simulink model "Waste_Classification"  (R2019a)
settings: Solver=FixedStepAuto  StartTime=0.0  StopTime=inf  FixedStep=0.002  RelTol=1e-3  EnableMultiTasking=on
undefined symbols (not defined in the file): height, HIL, left, qc_get_step_size, top, width
libraries: simulink x19, quarc_library x19
settings Model: SimulationMode=external  ExtModeTrigDuration=10000  Creator=dell  LastModifiedBy=郑怡迪
settings SolverCC: PositivePriorityOrder=on  AutoInsertRateTranBlk=on
settings RTWCC: SystemTargetFile=quarc_win64.tlc  TemplateMakefile=quarc_default_tmf  Description=QUARC Win64 Target
settings STFCustomTargetCC: TargetPreCompLibLocation=C:\PROGRA~3\QUARC\lib\2019a\win64\release  TargetLangStandard=C99 (ISO)  ConcurrentExecutionCompliant=on  SystemTargetFile=quarc_win64.tlc
settings GRTTargetCC: TargetPreCompLibLocation=C:\PROGRA~3\QUARC\lib\2019a\win64\release  ParMdlRefBuildCompliant=off  CompOptLevelCompliant=off  CombineOutputUpdateFcns=off  MatFileLogging=off  CPPClassGenCompliant=off  GRTInterface=on  UseToolchainInfoCompliant=off  ExtMode=on  ExtModeMexFile=quarc_comm

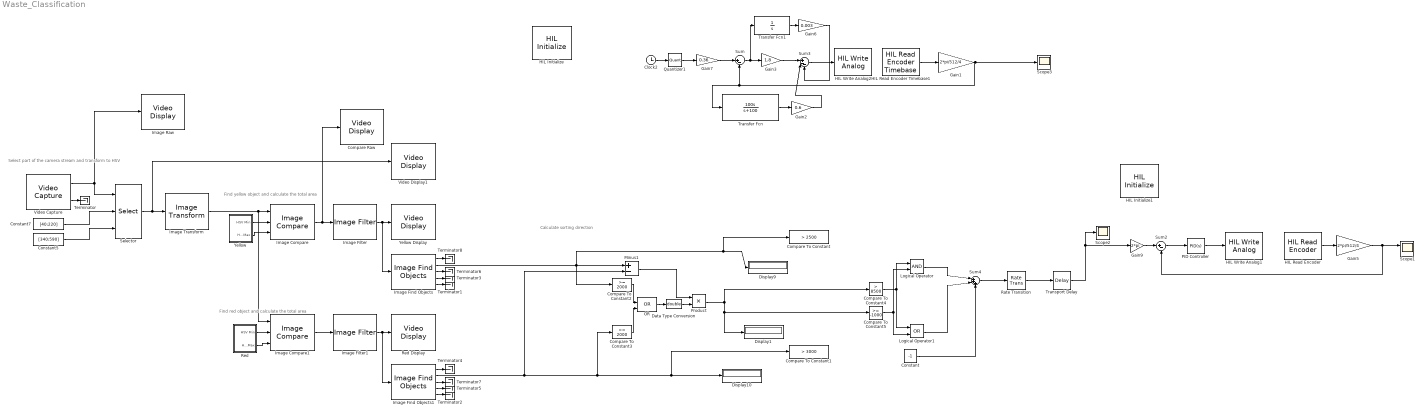
== system Waste_Classification ==
  note: Calculate sorting direction
  note: Find red object and calculate the total area
  note: Find yellow object and calculate the total area
  note: Select part of the camera stream and transform to HSV
  Clock2 : Clock
  Compare To Constant : simulink/Logic and Bit Operations/Compare To Constant  relop=>  const=2500  OutDataTypeStr=boolean
  Compare To Constant1 : simulink/Logic and Bit Operations/Compare To Constant  relop=>  const=3000  OutDataTypeStr=boolean
  Compare To Constant2 : simulink/Logic and Bit Operations/Compare To Constant  relop=>=  const=2000  OutDataTypeStr=boolean
  Compare To Constant3 : simulink/Logic and Bit Operations/Compare To Constant  relop=>=  const=2000  OutDataTypeStr=boolean
  Compare To Constant4 : simulink/Logic and Bit Operations/Compare To Constant  relop=>  const=8500  OutDataTypeStr=boolean
  Compare To Constant5 : simulink/Logic and Bit Operations/Compare To Constant  relop=>=  const=-1000  OutDataTypeStr=boolean
  Compare Raw : quarc_library/Multimedia/Video Display  Tag=slowlybeat6661/Compare Raw  sample_time=-1  use_hardware=on
  Constant : Constant  Value=-1
  Constant5 : Constant  Value=[340:590]
  Constant7 : Constant  Value=[40:220]
  Data Type Conversion : DataTypeConversion  OutDataTypeStr=double
  Display1 : Display
  Display10 : Display
  Display9 : Display
  Gain1 : Gain  Gain=2*pi/512/4
  Gain2 : Gain  Gain=0.6
  Gain3 : Gain  Gain=1.8
  Gain5 : Gain  Gain=2*pi/512/4
  Gain6 : Gain  Gain=0.003
  Gain7 : Gain  Gain=0.36
  Gain9 : Gain  Gain=2*pi
  HIL Initialize : quarc_library/Data Acquisition/Generic/Configuration/HIL Initialize  object_name=HIL-1  board_type=qube_servo2_usb  board_number=0  board_options=""  exclusive=off  active=on  hardware_clocks=[0]  clock_modes=[]  initial_clock_frequencies=[]  set_clock_params_at_start=off  set_clock_params_at_switch_in=off  set_clock_frequencies_at_start=off  set_clock_frequencies_at_switch_in=off  analog_input_channels=[0]  analog_input_configurations=[]  analog_input_maximums=3  analog_input_minimums=-3  set_analog_input_params_at_start=off  set_analog_input_params_at_switch_in=off  analog_output_channels=[0]  analog_output_maximums=15  analog_output_minimums=-15  initial_analog_outputs=[0]  final_analog_outputs=[0]  watchdog_analog_outputs=0  set_analog_output_params_at_start=off  set_analog_output_params_at_switch_in=off  set_analog_outputs_at_start=on  set_analog_outputs_at_switch_in=off  set_analog_outputs_at_terminate=on  set_analog_outputs_at_switch_out=off  set_analog_outputs_on_watchdog=on  digital_input_channels=[]  digital_output_channels=[0]  digital_output_configuration=[]  initial_digital_outputs=[1]  final_digital_outputs=[0]  watchdog_digital_outputs=[0]  set_digital_output_params_at_start=off  set_digital_output_params_at_switch_in=off  set_digital_outputs_at_start=on  set_digital_outputs_at_switch_in=off  set_digital_outputs_at_terminate=on  set_digital_outputs_at_switch_out=off  set_digital_outputs_on_watchdog=on  encoder_channels=[0:1]  quadrature=[4]  encoder_filter_frequency=[]  initial_encoder_counts=[0]  set_encoder_params_at_start=off  set_encoder_params_at_switch_in=off  set_encoder_counts_at_start=on  set_encoder_counts_at_switch_in=off  pwm_channels=[]  pwm_modes=[]  pwm_frequency=[]  pwm_configuration=[]  pwm_alignment=[]  pwm_polarity=[]  pwm_leading_deadband=[]  pwm_trailing_deadband=[]  initial_pwm_outputs=[]  final_pwm_outputs=[]  watchdog_pwm_outputs=[]  set_pwm_params_at_start=off  set_pwm_params_at_switch_in=off  set_pwm_outputs_at_start=off  set_pwm_outputs_at_switch_in=off  set_pwm_outputs_at_terminate=off  set_pwm_outputs_at_switch_out=off  set_pwm_outputs_on_watchdog=off  other_output_channels=[11000:11002]  initial_other_outputs=[0 1 0]  final_other_outputs=[1 0 0]  watchdog_other_outputs=[0 0 1]  set_other_outputs_at_start=on  set_other_outputs_at_switch_in=off  set_other_outputs_at_terminate=on  set_other_outputs_at_switch_out=off  set_other_outputs_on_watchdog=on
  HIL Initialize1 : quarc_library/Data Acquisition/Generic/Configuration/HIL Initialize  object_name=HIL-2  board_type=qube_servo2_usb  board_number=1  board_options=""  exclusive=off  active=on  hardware_clocks=[0]  clock_modes=[]  initial_clock_frequencies=[]  set_clock_params_at_start=off  set_clock_params_at_switch_in=off  set_clock_frequencies_at_start=off  set_clock_frequencies_at_switch_in=off  analog_input_channels=[0]  analog_input_configurations=[]  analog_input_maximums=3  analog_input_minimums=-3  set_analog_input_params_at_start=off  set_analog_input_params_at_switch_in=off  analog_output_channels=[0]  analog_output_maximums=15  analog_output_minimums=-15  initial_analog_outputs=[0]  final_analog_outputs=[0]  watchdog_analog_outputs=0  set_analog_output_params_at_start=off  set_analog_output_params_at_switch_in=off  set_analog_outputs_at_start=on  set_analog_outputs_at_switch_in=off  set_analog_outputs_at_terminate=on  set_analog_outputs_at_switch_out=off  set_analog_outputs_on_watchdog=on  digital_input_channels=[]  digital_output_channels=[0]  digital_output_configuration=[]  initial_digital_outputs=[1]  final_digital_outputs=[0]  watchdog_digital_outputs=[0]  set_digital_output_params_at_start=off  set_digital_output_params_at_switch_in=off  set_digital_outputs_at_start=on  set_digital_outputs_at_switch_in=off  set_digital_outputs_at_terminate=on  set_digital_outputs_at_switch_out=off  set_digital_outputs_on_watchdog=on  encoder_channels=[0:1]  quadrature=[4]  encoder_filter_frequency=[]  initial_encoder_counts=[0]  set_encoder_params_at_start=off  set_encoder_params_at_switch_in=off  set_encoder_counts_at_start=on  set_encoder_counts_at_switch_in=off  pwm_channels=[]  pwm_modes=[]  pwm_frequency=[]  pwm_configuration=[]  pwm_alignment=[]  pwm_polarity=[]  pwm_leading_deadband=[]  pwm_trailing_deadband=[]  initial_pwm_outputs=[]  final_pwm_outputs=[]  watchdog_pwm_outputs=[]  set_pwm_params_at_start=off  set_pwm_params_at_switch_in=off  set_pwm_outputs_at_start=off  set_pwm_outputs_at_switch_in=off  set_pwm_outputs_at_terminate=off  set_pwm_outputs_at_switch_out=off  set_pwm_outputs_on_watchdog=off  other_output_channels=[11000:11002]  initial_other_outputs=[0 1 0]  final_other_outputs=[1 0 0]  watchdog_other_outputs=[0 0 1]  set_other_outputs_at_start=on  set_other_outputs_at_switch_in=off  set_other_outputs_at_terminate=on  set_other_outputs_at_switch_out=off  set_other_outputs_on_watchdog=on
  HIL Read Encoder : quarc_library/Data Acquisition/Generic/Immediate I//O/HIL Read Encoder  object_name=HIL-2  channels=0  sample_time=qc_get_step_size  active=on  vector_output=off  data_type_mode=Inherit via back propagation  data_type=double
  HIL Read Encoder Timebase1 : quarc_library/Data Acquisition/Generic/Timebases/HIL Read Encoder Timebase  object_name=HIL-1  clock=0  channels=0  samples_in_buffer=max(ceil(1/qc_get_step_size), 1)  active=on  vector_output=off  data_type_mode=Inherit via back propagation  data_type=double
  HIL Write Analog1 : quarc_library/Data Acquisition/Generic/Immediate I//O/HIL Write Analog  object_name=HIL-2  channels=0  sample_time=-1  active=off  vector_input=off
  HIL Write Analog2 : quarc_library/Data Acquisition/Generic/Immediate I//O/HIL Write Analog  object_name=HIL-1  channels=0  sample_time=-1  active=off  vector_input=off
  Image Compare : quarc_library/Image Processing/Generic/Image Compare  output_type=Combined (one HxW output)  source=External input ports  r_comparison=min <= pixel and pixel <= max  r_minimum=0  r_maximum=16  g_comparison=min <= pixel and pixel <= max  g_minimum=128  g_maximum=255  b_comparison=min <= pixel and pixel <= max  b_minimum=64  b_maximum=255
      settings: SourceProductName=QUARC Targets
  Image Compare1 : quarc_library/Image Processing/Generic/Image Compare  output_type=Combined (one HxW output)  source=External input ports  r_comparison=min <= pixel and pixel <= max  r_minimum=0  r_maximum=16  g_comparison=min <= pixel and pixel <= max  g_minimum=128  g_maximum=255  b_comparison=min <= pixel and pixel <= max  b_minimum=64  b_maximum=255
      settings: SourceProductName=QUARC Targets
  Image Filter : quarc_library/Image Processing/Generic/Image Filter  filter_type=Depth hole-fill  source_of_roi=Internal dialog parameter  roi_style=[top, left, height, width]  roi=[]  maximum_roi=[]  roi_zone=Operate inside region of interest  border_type=Replicate  border_value=[0 0 0]  kernel_size=5  sigma=10  mask_size=[3 3]  kernel=int16([-2 -1 0; -1 1 1; 0 1 2])  divisor=1  offset=0  rounding=Nearest  algorithm_hint=None  threshold=100  alpha=0.9  num_frames=8  num_valid=1  gap_threshold=10  depth_threshold=255  iterations=2
      settings: AttributesFormatString=(%<filter_type>)  SourceProductName=QUARC Targets
  Image Filter1 : quarc_library/Image Processing/Generic/Image Filter  filter_type=Depth hole-fill  source_of_roi=Internal dialog parameter  roi_style=[top, left, height, width]  roi=[]  maximum_roi=[]  roi_zone=Operate inside region of interest  border_type=Replicate  border_value=[0 0 0]  kernel_size=5  sigma=10  mask_size=[3 3]  kernel=int16([-2 -1 0; -1 1 1; 0 1 2])  divisor=1  offset=0  rounding=Nearest  algorithm_hint=None  threshold=100  alpha=0.9  num_frames=8  num_valid=1  gap_threshold=10  depth_threshold=255  iterations=2
      settings: AttributesFormatString=(%<filter_type>)  SourceProductName=QUARC Targets
  Image Find Objects : quarc_library/Image Processing/Generic/Image Find Objects  num_objects=1  connectivity=4 directions (N, E, S, W)  sort_order=Sort by number of pixels  min_pixels=256  max_pixels=intmax('uint32')  largest=on  exclude_at_edges=off  variable_size=off  use_complex=off
      settings: SourceProductName=QUARC Targets
  Image Find Objects1 : quarc_library/Image Processing/Generic/Image Find Objects  num_objects=1  connectivity=4 directions (N, E, S, W)  sort_order=Sort by number of pixels  min_pixels=256  max_pixels=intmax('uint32')  largest=on  exclude_at_edges=off  variable_size=off  use_complex=off
      settings: SourceProductName=QUARC Targets
  Image Raw : quarc_library/Multimedia/Video Display  Tag=slowlybeat6661/Image Raw  sample_time=-1  use_hardware=on
  Image Transform : quarc_library/Image Processing/Generic/Image Transform  algorithm=RGB to HSV  color_theme=KRYGCBMW  min_pixel=0  max_pixel=4000
      settings: AttributesFormatString=(%<algorithm>)  SourceProductName=QUARC Targets
  Logical Operator : Logic  AllPortsSameDT=off  OutDataTypeStr=boolean
  Logical Operator1 : Logic  Operator=OR  AllPortsSameDT=off  OutDataTypeStr=boolean
  Minus1 : Sum  Inputs=+-  OutDataTypeStr=double
  OR : Logic  Operator=OR  IconShape=distinctive  AllPortsSameDT=off  OutDataTypeStr=boolean
  PID Controller : simulink/Continuous/PID Controller  Controller=PID  Form=Parallel  TimeDomain=Continuous-time  SampleTime=-1  IntegratorMethod=Forward Euler  FilterMethod=Forward Euler  ControllerParametersSource=internal  P=5  I=0.15  D=0.2  UseFilter=on  N=100  TunerSelectOption=Transfer Function Based (PID Tuner App)  InitialConditionSource=internal  InitialConditionForIntegrator=0  InitialConditionForFilter=0  DifferentiatorICPrevScaledInput=0  ExternalReset=none  TrackingMode=off  Kt=1  LimitOutput=off  UpperSaturationLimit=inf  LowerSaturationLimit=-inf  LinearizeAsGain=on  AntiWindupMode=none  Kb=1  POutMin=[]  POutMax=[]  IOutMin=[]  IOutMax=[]  DOutMin=[]  DOutMax=[]  NOutMin=[]  NOutMax=[]  SumOutMin=[]  SumOutMax=[]  SaturationOutMin=[]  SaturationOutMax=[]  PParamMin=[]  PParamMax=[]  IParamMin=[]  IParamMax=[]  DParamMin=[]  DParamMax=[]  NParamMin=[]  NParamMax=[]  KbParamMin=[]  KbParamMax=[]  KtParamMin=[]  KtParamMax=[]  KbOutMin=[]  KbOutMax=[]  KtOutMin=[]  KtOutMax=[]  IntegratorOutMin=[]  IntegratorOutMax=[]  FilterOutMin=[]  FilterOutMax=[]  SumI1OutMin=[]  SumI1OutMax=[]  SumI2OutMin=[]  SumI2OutMax=[]  SumI3OutMin=[]  SumI3OutMax=[]  SumI4OutMin=[]  SumI4OutMax=[]  SumDOutMin=[]  SumDOutMax=[]  DifferentiatorOutMin=[]  DifferentiatorOutMax=[]  FilterDiffOutCoefMin=[]  FilterDiffOutCoefMax=[]  ReciprocalOutMin=[]  ReciprocalOutMax=[]  SumDenOutMin=[]  SumDenOutMax=[]  SumNumOutMin=[]  SumNumOutMax=[]  DivideOutMin=[]  DivideOutMax=[]  IntegratorContinuousStateAttributes=''  IntegratorStateMustResolveToSignalObject=off  IntegratorRTWStateStorageClass=Auto  FilterContinuousStateAttributes=''  FilterStateMustResolveToSignalObject=off  FilterRTWStateStorageClass=Auto  ParallelPVariant=InternalParameters  IdealPVariant=Disabled  IVariant=InternalParameters  DVariant=InternalParameters  IntegratorVariant=Continuous  SatVariant=Disabled  AWVariant=Passthrough  PCopyVariant=Disabled  TRVariant=Disabled  FdbkBlocksVariant=Forward  IdealPFdbkVariant=Disabled  SatFdbkVariant=Disabled  DerivativeFilterVariant=ContFilter  NVariant=InternalParameters  NCopyVariant=Disabled  FilterICVariant=InternalICsFilter  IntegratorICVariant=InternalICs  ExternalResetVariant=Disabled  TRSumVariant=Passthrough  SumFdbkVariant=Disabled  SumVariant=Sum_PID
  Product : Product
  Quantizer1 : Quantizer
  Rate Transition : RateTransition
  Red : Subsystem
  Red Display : quarc_library/Multimedia/Video Display  Tag=slowlybeat6661/Red Display  sample_time=-1  use_hardware=on
  Scope1 : Scope  NumInputPorts=2
  Scope2 : Scope
  Scope3 : Scope
  Selector : Selector  NumberOfDimensions=3  IndexOptions=Index vector (port),Index vector (port),Select all  Indices=[1 3],1,1  OutputSizes=1,1,1
  Sum : Sum  Inputs=|+-
  Sum2 : Sum  Inputs=|+-
  Sum3 : Sum  Inputs=|+--
  Sum4 : Sum  Inputs=|+++
  Terminator{,1..8} (9 alike) : Terminator
  Transfer Fcn : TransferFcn  Numerator=[100 0]  Denominator=[1 100]
  Transfer Fcn1 : TransferFcn  Denominator=[1 0]
  Transport Delay : TransportDelay
  Video Capture : quarc_library/Multimedia/Video Capture  source=device  device=0  filename=sample_movie.mov  value=[0 0; 0 0]  resolution=640 x 480  width=640  height=480  output_format=MATLAB RGB (HxWx3)  data_type=uint8  sample_time=qc_get_step_size * ceil(0.033 / qc_get_step_size)  brightness_override=off  brightness=54.0  contrast_override=off  contrast=0.0  hue_override=off  hue=50.0  saturation_override=off  saturation=50  sharpness_override=off  sharpness=50.0  gamma_override=off  gamma=50.0  coloreffect_override=off  coloreffect=None  whitebalance_override=off  whitebalance=0.0  backlightcompensation_override=off  backlightcompensation=0.0  gain_override=off  gain=0.0  pan_override=off  pan=50.0  tilt_override=off  tilt=50.0  roll_override=off  roll=50.0  zoom_override=off  zoom=0.0  exposure_override=off  exposure=50.0  iris_override=off  iris=50.0  focus_override=off  focus=0.0
      settings: SourceProductName=QUARC Targets
  Video Display1 : quarc_library/Multimedia/Video Display  Tag=slowlybeat6661/Video Display1  sample_time=-1  use_hardware=on
  Yellow : Subsystem
  Yellow Display : quarc_library/Multimedia/Video Display  Tag=slowlybeat6661/Yellow Display  sample_time=-1  use_hardware=on
  wires:
  Gain5/1 -> Scope1/1, Sum2/2
  HIL Read Encoder/1 -> Gain5/1
  Product/1 -> Compare To Constant4/1, Compare To Constant5/1, Display1/1
  OR/1 -> Data Type Conversion/1
  Image Find Objects/1 -> Terminator8/1
  Constant7/1 -> Selector/2
  Video Capture/1 -> Image Raw/1, Selector/1
  Image Filter1/1 -> Image Find Objects1/1, Red Display/1
  Image Find Objects1/1 -> Terminator4/1
  Red/2(HSV Max) -> Image Compare1/3
  Image Find Objects1/2 -> Minus1/2, Display10/1, Compare To Constant1/1, Compare To Constant3/1
  Compare To Constant3/1 -> OR/2
  Selector/1 -> Video Display1/1, Image Transform/1
  Image Find Objects1/5 -> Terminator2/1
  Image Compare1/1 -> Image Filter1/1
  Yellow/2(HSV Max) -> Image Compare/3
  Image Compare/1 -> Image Filter/1, Compare Raw/1
  Image Find Objects/5 -> Terminator1/1
  Image Transform/1 -> Image Compare1/1, Image Compare/1
  Image Find Objects/4 -> Terminator3/1
  Image Filter/1 -> Yellow Display/1, Image Find Objects/1
  Image Find Objects1/3 -> Terminator7/1
  Video Capture/2 -> Terminator/1
  Image Find Objects/3 -> Terminator6/1
  Image Find Objects/2 -> Display9/1, Compare To Constant/1, Minus1/1, Compare To Constant2/1
  Image Find Objects1/4 -> Terminator5/1
  Data Type Conversion/1 -> Product/2
  Minus1/1 -> Product/1
  Red/1(HSV Min) -> Image Compare1/2
  Constant5/1 -> Selector/3
  Yellow/1(HSV Min) -> Image Compare/2
  Compare To Constant2/1 -> OR/1
  Compare To Constant4/1 -> Logical Operator1/1, Logical Operator/1
  Logical Operator/1 -> Sum4/1
  Logical Operator1/1 -> Sum4/2
  Constant/1 -> Sum4/3
  Sum4/1 -> Rate Transition/1
  Transport Delay/1 -> Scope2/1, Gain9/1
  Compare To Constant5/1 -> Logical Operator/2, Logical Operator1/2
  PID Controller/1 -> HIL Write Analog1/1
  Gain9/1 -> Sum2/1
  Sum2/1 -> PID Controller/1
  Gain7/1 -> Sum/1
  Quantizer1/1 -> Gain7/1
  Gain6/1 -> Sum3/3
  Clock2/1 -> Quantizer1/1
  Transfer Fcn1/1 -> Gain6/1
  Sum3/1 -> HIL Write Analog2/1
  Gain2/1 -> Sum3/2
  Transfer Fcn/1 -> Gain2/1
  Gain1/1 -> Scope3/1, Sum/2, Transfer Fcn/1
  Gain3/1 -> Sum3/1
  Sum/1 -> Gain3/1, Transfer Fcn1/1
  HIL Read Encoder Timebase1/1 -> Gain1/1
  Rate Transition/1 -> Transport Delay/1

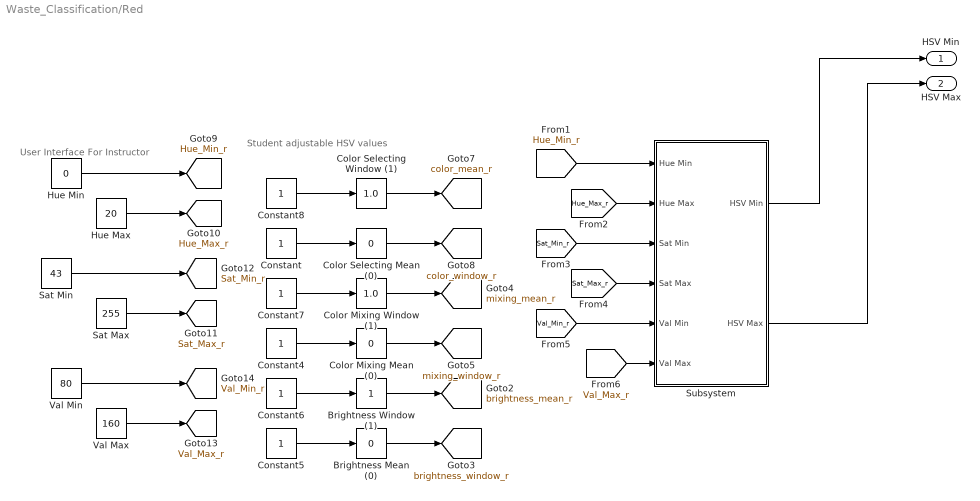
== system Waste_Classification/Red ==
  note: Student adjustable HSV values
  note: User Interface For Instructor
  Brightness Mean (0) : simulink/Math Operations/Slider Gain  gain=0  low=-1  high=1
  Brightness Window (1) : simulink/Math Operations/Slider Gain  gain=1  low=0  high=1
  Color Mixing Mean (0) : simulink/Math Operations/Slider Gain  gain=0  low=-1  high=1
  Color Mixing Window (1) : simulink/Math Operations/Slider Gain  gain=1.0  low=0  high=1
  Color Selecting Mean (0) : simulink/Math Operations/Slider Gain  gain=0  low=-1  high=1
  Color Selecting Window (1) : simulink/Math Operations/Slider Gain  gain=1.0  low=0  high=1
  Constant{,4..8} (6 alike) : Constant
  Hue Max : Constant  Value=20
  Hue Min : Constant  Value=0
  Sat Max : Constant  Value=255
  Sat Min : Constant  Value=43
  Subsystem : Subsystem
  Val Max : Constant  Value=160
  Val Min : Constant  Value=80
  HSV Min : Outport  VectorParamsAs1DForOutWhenUnconnected=on
  HSV Max : Outport  Port=2  VectorParamsAs1DForOutWhenUnconnected=on
  tag scope: Hue_Max_r=global, Hue_Min_r=global, Sat_Max_r=global, Sat_Min_r=global, Val_Max_r=global, Val_Min_r=global, brightness_mean_r=global, brightness_window_r=global, color_mean_r=global, color_window_r=global, mixing_mean_r=global, mixing_window_r=global
  wires:
  Subsystem/1(HSV Min) -> HSV Min/1
  Subsystem/2(HSV Max) -> HSV Max/1
  [Sat_Min_r] -> Subsystem/3(Sat Min)
  [Val_Max_r] -> Subsystem/6(Val Max)
  [Hue_Max_r] -> Subsystem/2(Hue Max)
  [Hue_Min_r] -> Subsystem/1(Hue Min)
  Color Mixing Window (1)/1 -> [mixing_mean_r]
  Constant6/1 -> Brightness Window (1)/1
  Constant4/1 -> Color Mixing Mean (0)/1
  Color Selecting Mean (0)/1 -> [color_window_r]
  [Val_Min_r] -> Subsystem/5(Val Min)
  Constant7/1 -> Color Mixing Window (1)/1
  Constant8/1 -> Color Selecting Window (1)/1
  Brightness Mean (0)/1 -> [brightness_window_r]
  Constant5/1 -> Brightness Mean (0)/1
  Hue Max/1 -> [Hue_Max_r]
  Constant/1 -> Color Selecting Mean (0)/1
  Brightness Window (1)/1 -> [brightness_mean_r]
  Sat Min/1 -> [Sat_Min_r]
  Color Selecting Window (1)/1 -> [color_mean_r]
  Sat Max/1 -> [Sat_Max_r]
  Color Mixing Mean (0)/1 -> [mixing_window_r]
  Val Min/1 -> [Val_Min_r]
  [Sat_Max_r] -> Subsystem/4(Sat Max)
  Val Max/1 -> [Val_Max_r]
  Hue Min/1 -> [Hue_Min_r]

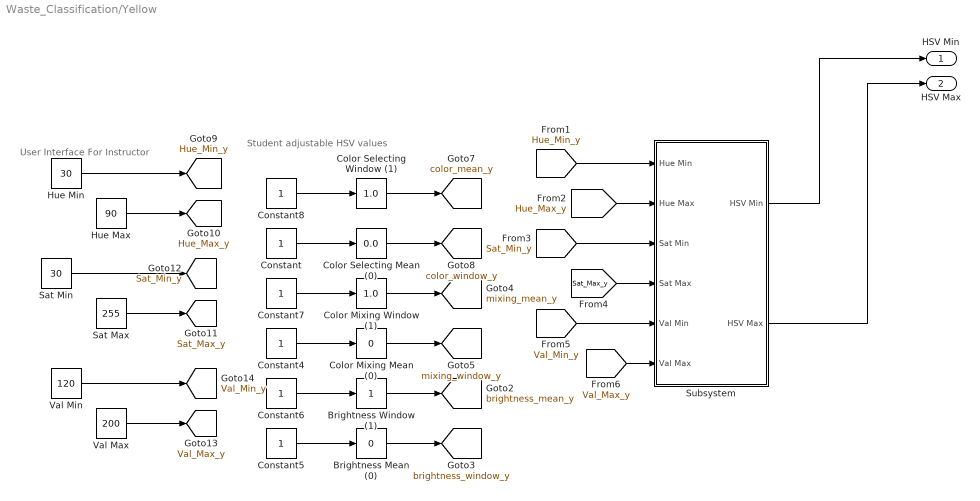
== system Waste_Classification/Yellow ==
  note: User Interface For Instructor
  note: Student adjustable HSV values
  Brightness Mean (0) : simulink/Math Operations/Slider Gain  gain=0  low=-1  high=1
  Brightness Window (1) : simulink/Math Operations/Slider Gain  gain=1  low=0  high=1
  Color Mixing Mean (0) : simulink/Math Operations/Slider Gain  gain=0  low=-1  high=1
  Color Mixing Window (1) : simulink/Math Operations/Slider Gain  gain=1.0  low=0  high=1
  Color Selecting Mean (0) : simulink/Math Operations/Slider Gain  gain=0.0  low=-1  high=1
  Color Selecting Window (1) : simulink/Math Operations/Slider Gain  gain=1.0  low=0  high=1
  Constant{,4..8} (6 alike) : Constant
  Hue Max : Constant  Value=90
  Hue Min : Constant  Value=30
  Sat Max : Constant  Value=255
  Sat Min : Constant  Value=30
  Subsystem : Subsystem
  Val Max : Constant  Value=200
  Val Min : Constant  Value=120
  HSV Min : Outport  VectorParamsAs1DForOutWhenUnconnected=on
  HSV Max : Outport  Port=2  VectorParamsAs1DForOutWhenUnconnected=on
  tag scope: Hue_Max_y=global, Hue_Min_y=global, Sat_Max_y=global, Sat_Min_y=global, Val_Max_y=global, Val_Min_y=global, brightness_mean_y=global, brightness_window_y=global, color_mean_y=global, color_window_y=global, mixing_mean_y=global, mixing_window_y=global
  wires:
  Hue Min/1 -> [Hue_Min_y]
  Val Max/1 -> [Val_Max_y]
  [Sat_Max_y] -> Subsystem/4(Sat Max)
  Val Min/1 -> [Val_Min_y]
  Color Mixing Mean (0)/1 -> [mixing_window_y]
  Sat Max/1 -> [Sat_Max_y]
  Color Selecting Window (1)/1 -> [color_mean_y]
  Sat Min/1 -> [Sat_Min_y]
  Brightness Window (1)/1 -> [brightness_mean_y]
  Constant/1 -> Color Selecting Mean (0)/1
  Hue Max/1 -> [Hue_Max_y]
  Constant5/1 -> Brightness Mean (0)/1
  Brightness Mean (0)/1 -> [brightness_window_y]
  Constant8/1 -> Color Selecting Window (1)/1
  Constant7/1 -> Color Mixing Window (1)/1
  [Val_Min_y] -> Subsystem/5(Val Min)
  Color Selecting Mean (0)/1 -> [color_window_y]
  Constant4/1 -> Color Mixing Mean (0)/1
  Constant6/1 -> Brightness Window (1)/1
  Color Mixing Window (1)/1 -> [mixing_mean_y]
  [Hue_Min_y] -> Subsystem/1(Hue Min)
  [Hue_Max_y] -> Subsystem/2(Hue Max)
  [Val_Max_y] -> Subsystem/6(Val Max)
  [Sat_Min_y] -> Subsystem/3(Sat Min)
  Subsystem/2(HSV Max) -> HSV Max/1
  Subsystem/1(HSV Min) -> HSV Min/1

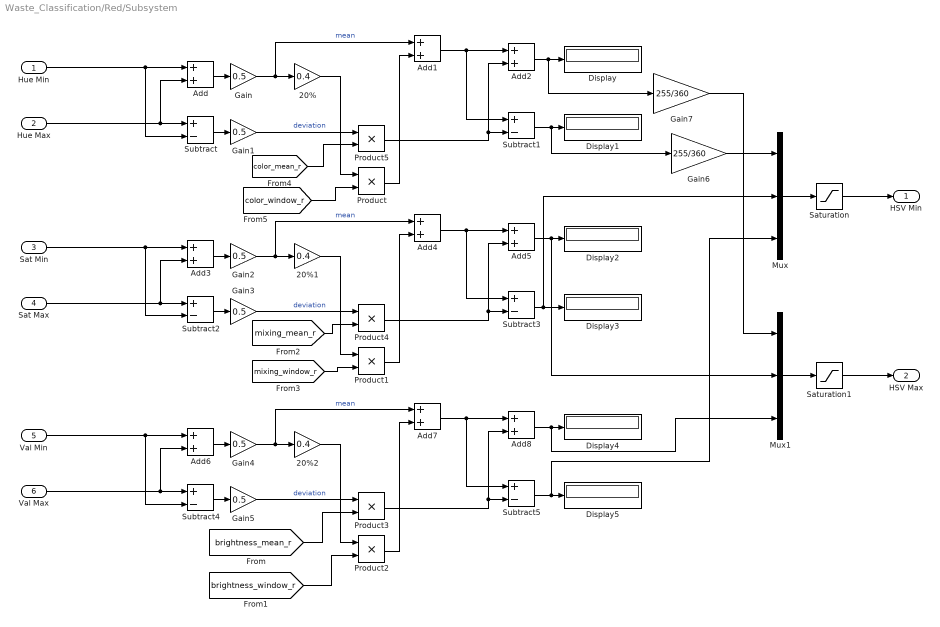
== system Waste_Classification/Red/Subsystem ==
  Hue Min : Inport
  Hue Max : Inport  Port=2
  Sat Min : Inport  Port=3
  Sat Max : Inport  Port=4
  Val Min : Inport  Port=5
  Val Max : Inport  Port=6
  20% : Gain  Gain=0.4
  20%1 : Gain  Gain=0.4
  20%2 : Gain  Gain=0.4
  Add{,1..8} (9 alike) : Sum
  Display{,1..5} (6 alike) : Display
  Gain{,1..5} (6 alike) : Gain  Gain=0.5
  Gain6 : Gain  Gain=255/360
  Gain7 : Gain  Gain=255/360
  Mux : Mux  Inputs=3
  Mux1 : Mux  Inputs=3
  Product{,1..5} (6 alike) : Product
  Saturation : Saturate  UpperLimit=[255 255 255]  LowerLimit=[0 0 0]
  Saturation1 : Saturate  UpperLimit=[255 255 255]  LowerLimit=[0 0 0]
  Subtract{,1..5} (6 alike) : Sum  Inputs=+-
  HSV Min : Outport
  HSV Max : Outport  Port=2
  wires:
  Product1/1 -> Add4/2
  Val Min/1 -> Add6/1, Subtract4/2
  Mux/1 -> Saturation/1
  Subtract1/1 -> Gain6/1, Display1/1
  Subtract4/1 -> Gain5/1
  Add1/1 -> Subtract1/1, Add2/1
  Product3/1 -> Add8/2, Subtract5/2
  Product2/1 -> Add7/2
  Gain4/1 -> 20%2/1, Add7/1  "mean"
  Add2/1 -> Gain7/1, Display/1
  Subtract3/1 -> Mux/2, Display3/1
  Subtract5/1 -> Mux/3, Display5/1
  Gain/1 -> 20%/1, Add1/1  "mean"
  Sat Min/1 -> Subtract2/2, Add3/1
  Subtract2/1 -> Gain3/1
  Product5/1 -> Add2/2, Subtract1/2
  Gain5/1 -> Product3/1  "deviation"
  Add5/1 -> Mux1/2, Display2/1
  Gain2/1 -> Add4/1, 20%1/1  "mean"
  Add8/1 -> Mux1/3, Display4/1
  Product/1 -> Add1/2
  Subtract/1 -> Gain1/1
  Product4/1 -> Subtract3/2, Add5/2
  Add4/1 -> Add5/1, Subtract3/1
  Add7/1 -> Subtract5/1, Add8/1
  Sat Max/1 -> Subtract2/1, Add3/2
  20%1/1 -> Product1/1
  [brightness_mean_r] -> Product3/2
  Mux1/1 -> Saturation1/1
  Add3/1 -> Gain2/1
  [mixing_mean_r] -> Product4/2
  Hue Min/1 -> Add/1, Subtract/2
  Hue Max/1 -> Add/2, Subtract/1
  Gain3/1 -> Product4/1  "deviation"
  Val Max/1 -> Add6/2, Subtract4/1
  20%2/1 -> Product2/1
  Add6/1 -> Gain4/1
  [color_window_r] -> Product/2
  [color_mean_r] -> Product5/2
  20%/1 -> Product/1
  Add/1 -> Gain/1
  Gain1/1 -> Product5/1  "deviation"
  [mixing_window_r] -> Product1/2
  [brightness_window_r] -> Product2/2
  Saturation/1 -> HSV Min/1
  Saturation1/1 -> HSV Max/1
  Gain6/1 -> Mux/1
  Gain7/1 -> Mux1/1

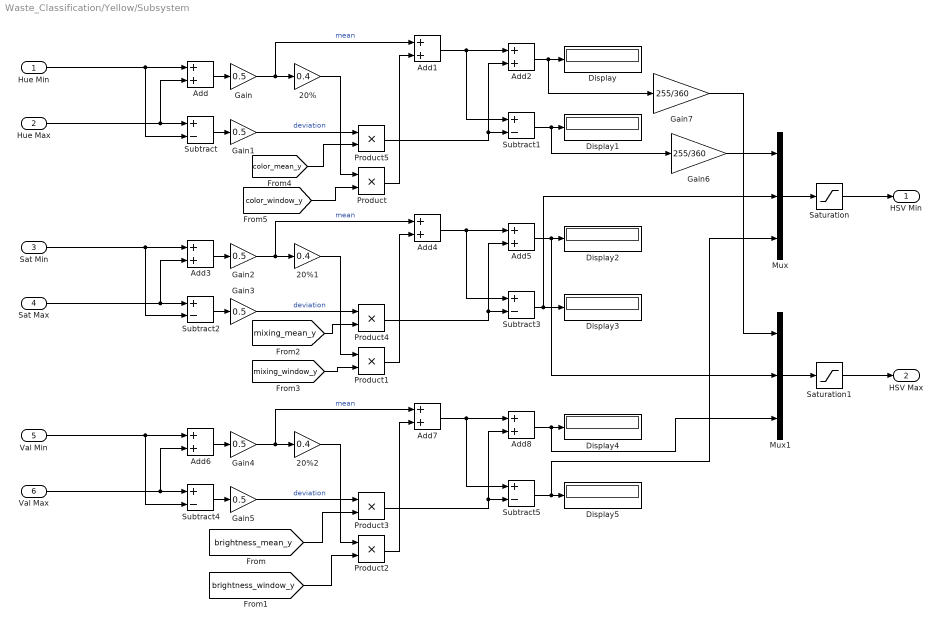
== system Waste_Classification/Yellow/Subsystem ==
  Hue Min : Inport
  Hue Max : Inport  Port=2
  Sat Min : Inport  Port=3
  Sat Max : Inport  Port=4
  Val Min : Inport  Port=5
  Val Max : Inport  Port=6
  20% : Gain  Gain=0.4
  20%1 : Gain  Gain=0.4
  20%2 : Gain  Gain=0.4
  Add{,1..8} (9 alike) : Sum
  Display{,1..5} (6 alike) : Display
  Gain{,1..5} (6 alike) : Gain  Gain=0.5
  Gain6 : Gain  Gain=255/360
  Gain7 : Gain  Gain=255/360
  Mux : Mux  Inputs=3
  Mux1 : Mux  Inputs=3
  Product{,1..5} (6 alike) : Product
  Saturation : Saturate  UpperLimit=[255 255 255]  LowerLimit=[0 0 0]
  Saturation1 : Saturate  UpperLimit=[255 255 255]  LowerLimit=[0 0 0]
  Subtract{,1..5} (6 alike) : Sum  Inputs=+-
  HSV Min : Outport
  HSV Max : Outport  Port=2
  wires:
  Gain7/1 -> Mux1/1
  Gain6/1 -> Mux/1
  Saturation1/1 -> HSV Max/1
  Saturation/1 -> HSV Min/1
  [brightness_window_y] -> Product2/2
  [mixing_window_y] -> Product1/2
  Gain1/1 -> Product5/1  "deviation"
  Add/1 -> Gain/1
  20%/1 -> Product/1
  [color_mean_y] -> Product5/2
  [color_window_y] -> Product/2
  Add6/1 -> Gain4/1
  20%2/1 -> Product2/1
  Val Max/1 -> Subtract4/1, Add6/2
  Gain3/1 -> Product4/1  "deviation"
  Hue Max/1 -> Subtract/1, Add/2
  Hue Min/1 -> Subtract/2, Add/1
  [mixing_mean_y] -> Product4/2
  Add3/1 -> Gain2/1
  Mux1/1 -> Saturation1/1
  [brightness_mean_y] -> Product3/2
  20%1/1 -> Product1/1
  Sat Max/1 -> Add3/2, Subtract2/1
  Add7/1 -> Add8/1, Subtract5/1
  Add4/1 -> Subtract3/1, Add5/1
  Product4/1 -> Add5/2, Subtract3/2
  Subtract/1 -> Gain1/1
  Product/1 -> Add1/2
  Add8/1 -> Display4/1, Mux1/3
  Gain2/1 -> 20%1/1, Add4/1  "mean"
  Add5/1 -> Display2/1, Mux1/2
  Gain5/1 -> Product3/1  "deviation"
  Product5/1 -> Subtract1/2, Add2/2
  Subtract2/1 -> Gain3/1
  Sat Min/1 -> Add3/1, Subtract2/2
  Gain/1 -> Add1/1, 20%/1  "mean"
  Subtract5/1 -> Display5/1, Mux/3
  Subtract3/1 -> Display3/1, Mux/2
  Add2/1 -> Display/1, Gain7/1
  Gain4/1 -> Add7/1, 20%2/1  "mean"
  Product2/1 -> Add7/2
  Product3/1 -> Subtract5/2, Add8/2
  Add1/1 -> Add2/1, Subtract1/1
  Subtract4/1 -> Gain5/1
  Subtract1/1 -> Display1/1, Gain6/1
  Mux/1 -> Saturation/1
  Val Min/1 -> Subtract4/2, Add6/1
  Product1/1 -> Add4/2
